simulink model "Servo_Disturbance_Rejection_with_observ"  (R2017a)
settings: Solver=VariableStepAuto  StartTime=0.0  StopTime=50  FixedStep=0.01  RelTol=1e-3  EnableMultiTasking=on
values from neighbouring files (symbols this model uses):
  A = [A11 A12; A21 A22]    [buck_boost_sys_define.m]
  AObs = A-L*C    [make_graphs.m]    (also in servo_observ.m)
  B = [(Vin+X2)/L; -X1/C]    [buck_boost_sys_define.m]
  BObs = [B , L]    [make_graphs.m]    (also in servo_observ.m)
  C = [0 1]    [buck_boost_sys_define.m]
  CObs = eye(2)    [make_graphs.m]    (also in servo_observ.m)
  D = [0]    [buck_boost_sys_define.m]
  DObs = zeros(2,2)    [make_graphs.m]    (also in servo_observ.m)
  Gc = 1/(C*(B*Kt-A)^-1*B)    [make_graphs.m]    (also in servo_observ.m)
  K = Ksrv(j,1:2)    [make_graphs.m]    (also in servo_observ.m = Ksrv(1:2))
  ki = - Ksrv(j,3)    [make_graphs.m]    (also in servo_observ.m = - Ksrv(3))
  Kt = place(A,B,desP_track)    [make_graphs.m]    (also in servo_observ.m)
  U = 0.5    [buck_boost_sys_define.m]
  x0 = [0 0]'    [make_graphs.m]    (also in servo_observ.m)
  x0_hat = [0, 0]'    [make_graphs.m]    (also in servo_observ.m)
  X1 = Vin*U/((U-1)*(U-1)*R)    (= 0.0196078431373)    [buck_boost_sys_define.m]
  X2 = Vin*U/(1-U)    (= 5)    [buck_boost_sys_define.m]
libraries: simulink x1
settings Model: Creator=Bara  LastModifiedBy=loreliegordon
settings OptimizationCC: LifeSpan=inf
settings DebuggingCC: SFUnexpectedBacktrackingDiag=warning  SFNoUnconditionalDefaultTransitionDiag=warning  SFExecutionAtInitializationDiag=none
settings GRTTargetCC: TargetLangStandard=C89/C90 (ANSI)  GeneratePreprocessorConditionals=Disable all
settings ConfigComp: CovMetricSettings=dw  CovHtmlReporting=on  CovSaveCumulativeToWorkspaceVar=on  CovSaveSingleToWorkspaceVar=on  CovExternalEMLEnable=off

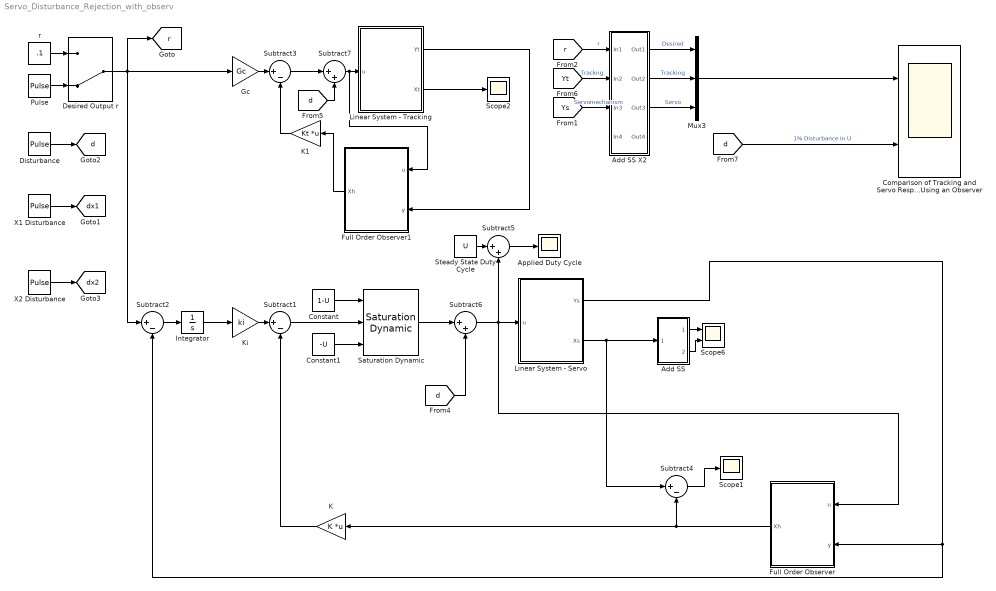
== system Servo_Disturbance_Rejection_with_observ ==
  Add SS : Subsystem
  Add SS X2 : Subsystem
  Applied Duty Cycle : Scope
  Comparison of Tracking and Servo Response Systems Using an Observer : Scope  NumInputPorts=2
  Constant : Constant  Value=1-U
  Constant1 : Constant  Value=-U
  Desired Output r : ManualSwitch  CurrentSetting=0
  Disturbance : DiscretePulseGenerator  PulseType=Time based  Amplitude=0.01  Period=20  PulseWidth=25  PhaseDelay=2.5
  Full Order Observer : Subsystem
  Full Order Observer1 : Subsystem
  Gc : Gain  Gain=Gc
  Integrator : Integrator  InitialCondition=C*x0
  K : Gain  Gain=K  Multiplication=Matrix(K*u) (u vector)
  K1 : Gain  Gain=Kt  Multiplication=Matrix(K*u) (u vector)
  Ki : Gain  Gain=ki
  Linear System - Servo : Subsystem
  Linear System - Tracking : Subsystem
  Mux3 : Mux  Inputs=3
  Pulse : DiscretePulseGenerator  PulseType=Time based  Period=40  PulseWidth=50
  Saturation Dynamic : simulink/Discontinuities/Saturation Dynamic  OutMin=[]  OutMax=[]  OutDataTypeStr=Inherit: Same as second input  OutDataType=fixdt(1, 16)  OutScaling=2^-10  DoSatur=off
  Scope1 : Scope
  Scope2 : Scope
  Scope6 : Scope  NumInputPorts=2
  Steady State Duty Cycle : Constant  Value=U
  Subtract{1..4} (4 alike) : Sum  Inputs=|+-
  Subtract5 : Sum  Inputs=|++
  Subtract6 : Sum  Inputs=|++
  Subtract7 : Sum  Inputs=|++
  X1 Disturbance : DiscretePulseGenerator  PulseType=Time based  Amplitude=.01*U  Period=20  PulseWidth=25  PhaseDelay=12.5
  X2 Disturbance : DiscretePulseGenerator  PulseType=Time based  Amplitude=0.0  Period=20  PulseWidth=25  PhaseDelay=2.5
  r : Constant  Value=.1
  tag scope: d=global, dx1=global, dx2=global, r=global
  wires:
  Mux3/1 -> Comparison of Tracking and Servo Response Systems Using an Observer/1
  [Ys] -> Add SS X2/3(In3)  "Servomechanism"
  r/1 -> Desired Output r/1
  Pulse/1 -> Desired Output r/2
  K/1 -> Subtract1/2
  Ki/1 -> Subtract1/1
  Integrator/1 -> Ki/1
  Subtract2/1 -> Integrator/1
  Linear System - Servo/1(Ys) -> Full Order Observer/2(y), Subtract2/2
  Disturbance/1 -> [d]
  Linear System - Tracking/2(Xt) -> Scope2/1
  K1/1 -> Subtract3/2
  Gc/1 -> Subtract3/1
  Desired Output r/1 -> Gc/1, [r], Subtract2/1
  Constant/1 -> Saturation Dynamic/1
  Constant1/1 -> Saturation Dynamic/3
  Linear System - Servo/2(Xs) -> Subtract4/1, Add SS/1(In1)
  X1 Disturbance/1 -> [dx1]
  X2 Disturbance/1 -> [dx2]
  Add SS X2/3(Out3) -> Mux3/3  "Servo"
  [Yt] -> Add SS X2/2(In2)  "Trackng"
  Add SS X2/2(Out2) -> Mux3/2  "Tracking"
  [r] -> Add SS X2/1(In1)  "r"
  Add SS X2/1(Out1) -> Mux3/1  "Desired"
  Add SS/1(Out1) -> Scope6/1
  Add SS/2(Out2) -> Scope6/2
  Subtract5/1 -> Applied Duty Cycle/1
  Steady State Duty Cycle/1 -> Subtract5/1
  Full Order Observer/1(Xh) -> Subtract4/2, K/1
  Subtract4/1 -> Scope1/1
  Subtract6/1 -> Full Order Observer/1(u), Subtract5/2, Linear System - Servo/1(u)
  [d] -> Subtract6/2
  [d] -> Subtract7/2
  Subtract3/1 -> Subtract7/1
  Subtract7/1 -> Full Order Observer1/1(u), Linear System - Tracking/1(u)
  Linear System - Tracking/1(Yt) -> Full Order Observer1/2(y)
  Full Order Observer1/1(Xh) -> K1/1
  Subtract1/1 -> Saturation Dynamic/2
  Saturation Dynamic/1 -> Subtract6/1
  [d] -> Comparison of Tracking and Servo Response Systems Using an Observer/2  "1% Disturbance in U"

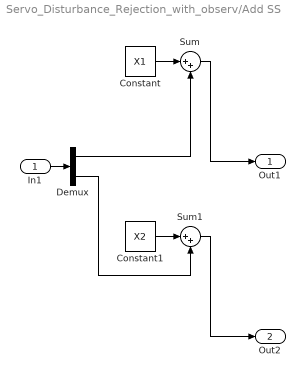
== system Servo_Disturbance_Rejection_with_observ/Add SS ==
  In1 : Inport
  Constant : Constant  Value=X1
  Constant1 : Constant  Value=X2
  Demux : Demux  Outputs=2
  Sum : Sum  Inputs=|++
  Sum1 : Sum  Inputs=|++
  Out1 : Outport
  Out2 : Outport  Port=2
  wires:
  Constant1/1 -> Sum1/1
  Sum/1 -> Out1/1
  Constant/1 -> Sum/1
  Demux/1 -> Sum/2
  Demux/2 -> Sum1/2
  Sum1/1 -> Out2/1
  In1/1 -> Demux/1

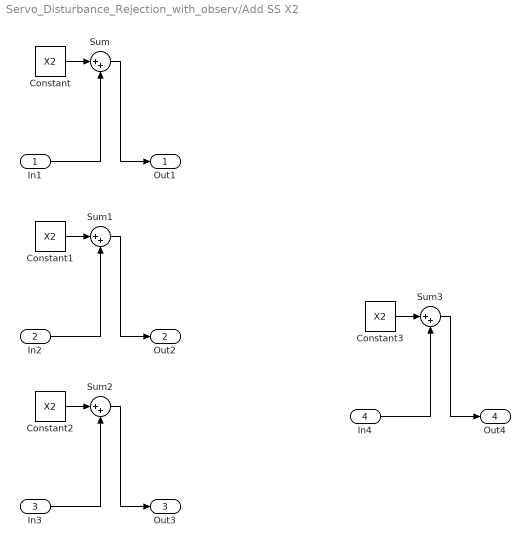
== system Servo_Disturbance_Rejection_with_observ/Add SS X2 ==
  In1 : Inport
  In2 : Inport  Port=2
  In3 : Inport  Port=3
  In4 : Inport  Port=4
  Constant{,1..3} (4 alike) : Constant  Value=X2
  Sum{,1..3} (4 alike) : Sum  Inputs=|++
  Out1 : Outport
  Out2 : Outport  Port=2
  Out3 : Outport  Port=3
  Out4 : Outport  Port=4
  wires:
  Sum/1 -> Out1/1
  In1/1 -> Sum/2
  Constant/1 -> Sum/1
  Constant1/1 -> Sum1/1
  Sum1/1 -> Out2/1
  In2/1 -> Sum1/2
  Constant2/1 -> Sum2/1
  Sum2/1 -> Out3/1
  In3/1 -> Sum2/2
  Sum3/1 -> Out4/1
  Constant3/1 -> Sum3/1
  In4/1 -> Sum3/2

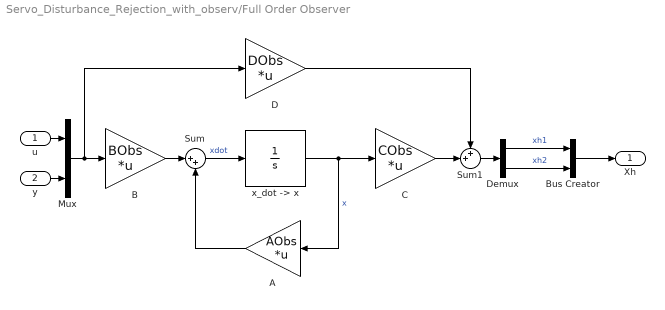
== system Servo_Disturbance_Rejection_with_observ/Full Order Observer ==
  u : Inport
  y : Inport  Port=2
  A : Gain  Gain=AObs  Multiplication=Matrix(K*u) (u vector)
  B : Gain  Gain=BObs  Multiplication=Matrix(K*u) (u vector)
  Bus Creator : BusCreator  Inputs=2
  C : Gain  Gain=CObs  Multiplication=Matrix(K*u) (u vector)
  D : Gain  Gain=DObs  Multiplication=Matrix(K*u) (u vector)
  Demux : Demux  Outputs=2
  Mux : Mux  Inputs=2
  Sum : Sum  Inputs=|++
  Sum1 : Sum  Inputs=++|
  "x_dot -> x" : Integrator  InitialCondition=x0_hat
  Xh : Outport
  wires:
  Sum/1 -> "x_dot -> x"/1  "xdot"
  "x_dot -> x"/1 -> A/1, C/1  "x"
  A/1 -> Sum/2
  B/1 -> Sum/1
  Mux/1 -> D/1, B/1
  C/1 -> Sum1/2
  D/1 -> Sum1/1
  Demux/1 -> Bus Creator/1  "xh1"
  Demux/2 -> Bus Creator/2  "xh2"
  Bus Creator/1 -> Xh/1
  u/1 -> Mux/1
  y/1 -> Mux/2
  Sum1/1 -> Demux/1

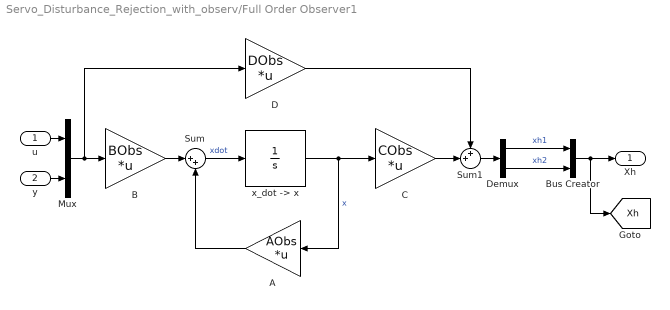
== system Servo_Disturbance_Rejection_with_observ/Full Order Observer1 ==
  u : Inport
  y : Inport  Port=2
  A : Gain  Gain=AObs  Multiplication=Matrix(K*u) (u vector)
  B : Gain  Gain=BObs  Multiplication=Matrix(K*u) (u vector)
  Bus Creator : BusCreator  Inputs=2
  C : Gain  Gain=CObs  Multiplication=Matrix(K*u) (u vector)
  D : Gain  Gain=DObs  Multiplication=Matrix(K*u) (u vector)
  Demux : Demux  Outputs=2
  Mux : Mux  Inputs=2
  Sum : Sum  Inputs=|++
  Sum1 : Sum  Inputs=++|
  "x_dot -> x" : Integrator  InitialCondition=x0_hat
  Xh : Outport
  tag scope: Xh=global
  wires:
  Sum1/1 -> Demux/1
  y/1 -> Mux/2
  u/1 -> Mux/1
  Bus Creator/1 -> [Xh], Xh/1
  Demux/2 -> Bus Creator/2  "xh2"
  Demux/1 -> Bus Creator/1  "xh1"
  D/1 -> Sum1/1
  C/1 -> Sum1/2
  Mux/1 -> B/1, D/1
  B/1 -> Sum/1
  A/1 -> Sum/2
  "x_dot -> x"/1 -> C/1, A/1  "x"
  Sum/1 -> "x_dot -> x"/1  "xdot"

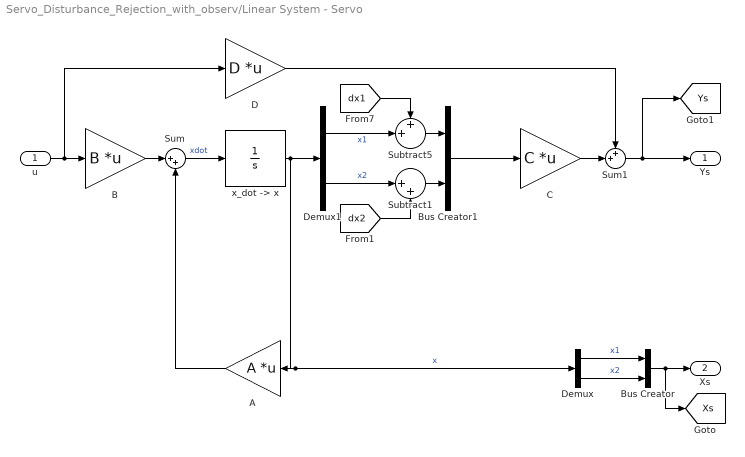
== system Servo_Disturbance_Rejection_with_observ/Linear System - Servo ==
  u : Inport
  A : Gain  Gain=A  Multiplication=Matrix(K*u) (u vector)
  B : Gain  Gain=B  Multiplication=Matrix(K*u) (u vector)
  Bus Creator : BusCreator  Inputs=2
  Bus Creator1 : BusCreator  Inputs=2
  C : Gain  Gain=C  Multiplication=Matrix(K*u) (u vector)
  D : Gain  Gain=D  Multiplication=Matrix(K*u) (u vector)
  Demux : Demux  Outputs=2
  Demux1 : Demux  Outputs=2
  Subtract1 : Sum  Inputs=|++
  Subtract5 : Sum  Inputs=++|
  Sum : Sum  Inputs=|++
  Sum1 : Sum  Inputs=++|
  "x_dot -> x" : Integrator  InitialCondition=x0
  Ys : Outport
  Xs : Outport  Port=2
  tag scope: Xs=global, Ys=global
  wires:
  Bus Creator/1 -> [Xs], Xs/1
  Demux/2 -> Bus Creator/2  "x2"
  Demux/1 -> Bus Creator/1  "x1"
  Sum1/1 -> Ys/1, [Ys]
  D/1 -> Sum1/1
  C/1 -> Sum1/2
  u/1 -> B/1, D/1
  B/1 -> Sum/1
  A/1 -> Sum/2
  "x_dot -> x"/1 -> Demux/1, A/1, Demux1/1  "x"
  Sum/1 -> "x_dot -> x"/1  "xdot"
  [dx1] -> Subtract5/1
  Demux1/1 -> Subtract5/2  "x1"
  Bus Creator1/1 -> C/1
  Subtract5/1 -> Bus Creator1/1
  Subtract1/1 -> Bus Creator1/2
  Demux1/2 -> Subtract1/1  "x2"
  [dx2] -> Subtract1/2

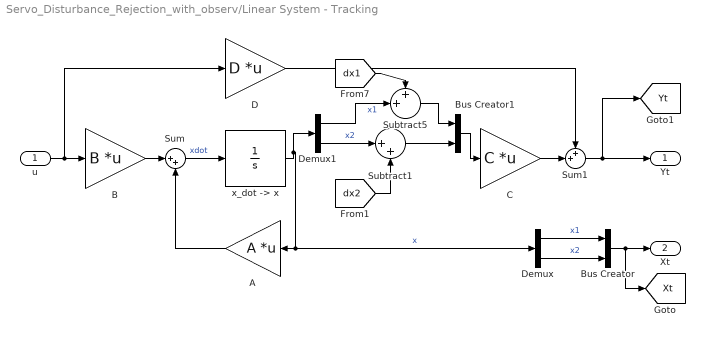
== system Servo_Disturbance_Rejection_with_observ/Linear System - Tracking ==
  u : Inport
  A : Gain  Gain=A  Multiplication=Matrix(K*u) (u vector)
  B : Gain  Gain=B  Multiplication=Matrix(K*u) (u vector)
  Bus Creator : BusCreator  Inputs=2
  Bus Creator1 : BusCreator  Inputs=2
  C : Gain  Gain=C  Multiplication=Matrix(K*u) (u vector)
  D : Gain  Gain=D  Multiplication=Matrix(K*u) (u vector)
  Demux : Demux  Outputs=2
  Demux1 : Demux  Outputs=2
  Subtract1 : Sum  Inputs=|++
  Subtract5 : Sum  Inputs=++|
  Sum : Sum  Inputs=|++
  Sum1 : Sum  Inputs=++|
  "x_dot -> x" : Integrator  InitialCondition=x0
  Yt : Outport
  Xt : Outport  Port=2
  tag scope: Xt=global, Yt=global
  wires:
  Sum/1 -> "x_dot -> x"/1  "xdot"
  A/1 -> Sum/2
  B/1 -> Sum/1
  u/1 -> D/1, B/1
  C/1 -> Sum1/2
  D/1 -> Sum1/1
  Sum1/1 -> [Yt], Yt/1
  Demux/1 -> Bus Creator/1  "x1"
  Demux/2 -> Bus Creator/2  "x2"
  Bus Creator/1 -> Xt/1, [Xt]
  [dx2] -> Subtract1/2
  "x_dot -> x"/1 -> Demux/1, A/1, Demux1/1  "x"
  Subtract5/1 -> Bus Creator1/1
  Demux1/1 -> Subtract5/2  "x1"
  Demux1/2 -> Subtract1/1  "x2"
  Subtract1/1 -> Bus Creator1/2
  [dx1] -> Subtract5/1
  Bus Creator1/1 -> C/1
